simulink model "interpolation_cubique"  (R2017b)
settings: Solver=FixedStepDiscrete  StartTime=0.0  StopTime=1  RelTol=1e-3
model workspace (MAT data in the model file):
  bande_passante = 20000000
  binary_sample_time = 2.51968503937e-08
  display = [0+0i 0+0i 0+0i 0+0i 0+0i 0+0i 0+0i 0+0i 0+0i 0+0i 0+0i 0+0i ... (40000 elements, 200x200)]
  nbr_pilote = 3
  nbr_sous_porteuse = 508
  nbr_total_canaux = 512
  nbr_zero = 1
  size_prefixe_cyclique = 3
  symbol_sample_time = 2.56e-05
  v = [0+0i; 0+0i; 0+0i; 0+0i; 0+0i; 0+0i; 0+0i; 0+0i; 0+0i; 0+0i; 0+0i; 0+0i; 0+0i; 0+0i; 0+0i; 0+0i; 0+0i; 0+0i; 0+0i; 0+0i; 0+0i; 0+0i; 0+0i; 0+0i; 0+0i; 0+0i; 0+0i; 0+0i; 0+0i; 0+0i; 0+0i; 0+0i; 0+0i; 0+0i; 0+0i; 0+0i; 0+0i; 0+0i; 0+0i; 0+0i; 0+0i; 0+0i; 0+0i; 0+0i; 0+0i; 0+0i; 0+0i; 0+0i; 0+0i; 0+0i; 0+0i; 0+0i; 0+0i; 0+0i; 0+0i; 0+0i; 0+0i; 0+0i; 0+0i; 0+0i; 0+0i; 0+0i; 0+0i; 0+0i; 0+0i; 0+0i; 0+0i; 0+0i; 0+0i; 0+0i; 0+0i; 0+0i; 0+0i; 0+0i; 0+0i; 0+0i; 0+0i; 0+0i; 0+0i; 0+0i; 0+0i; 0+0i; 0+0i; 0+0i; 0+0i; 0+0i; 0+0i; 0+0i; 0+0i; 0+0i; 0+0i; 0+0i; 0+0i; 0+0i; 0+0i; 0+0i; 0+0i; 0+0i; 0+0i; 0+0i; 0+0i; 0+0i; 0+0i; 0+0i; 0+0i; 0+0i; 0+0i; 0+0i; 0+0i; 0+0i; 0+0i; 0+0i; 0+0i; 0+0i; 0+0i; 0+0i; 0+0i; 0+0i; 0+0i; 0+0i; 0+0i; 0+0i; 0+0i; 0+0i; 0+0i; 0+0i; 0+0i; 0+0i; 0+0i; 0+0i; 0+0i; 0+0i; 0+0i; 0+0i; 0+0i; 0+0i; 0+0i; 0+0i; 0+0i; 0+0i; 0+0i; 0+0i; 0+0i; 0+0i; 0+0i; 0+0i; 0+0i; 0+0i; 0+0i; 0+0i; 0+0i; 0+0i; 0+0i; 0+0i; 0+0i; 0+0i; 0+0i; 0+0i; 0+0i; 0+0i; 0+0i; 0+0i; 0+0i; 0+0i; 0+0i; 0+0i; 0+0i; 0+0i; 0+0i; 0+0i; 0+0i; 0+0i; 0+0i; 0+0i; 0+0i; 0+0i; 0+0i; 0+0i; 0+0i; 0+0i; 0+0i; 0+0i; 0+0i; 0+0i; 0+0i; 0+0i; 0+0i; 0+0i; 0+0i; 0+0i; 0+0i; 0+0i; 0+0i; 0+0i; 0+0i; 0+0i; 0+0i; 0+0i; 0+0i; 0+0i; 0+0i; 0+0i; 0+0i; 0+0i; 0+0i; 0+0i; 0+0i; 0+0i; 0+0i; 0+0i; 0+0i; 0+0i; 0+0i; 0+0i; 0+0i; 0+0i; 0+0i; 0+0i; 0+0i; 0+0i; 0+0i; 0+0i; 0+0i; 0+0i; 0+0i; 0+0i; 0+0i; 0+0i; 0+0i; 0+0i; 0+0i; 0+0i; 0+0i; 0+0i; 0+0i; 0+0i; 0+0i; 0+0i; 0+0i; 0+0i; 0+0i; 0+0i; 0+0i; 0+0i; 0+0i; 0+0i; 0+0i; 0+0i; 0+0i; 0+0i; 0+0i; 0+0i; 0+0i; 0+0i; 0+0i; 0+0i]
values from neighbouring files (symbols this model uses):
  interval_pilote = 150    [workspace.m]
undefined symbols (not defined in the file or in its folder): doppler
libraries: commchan3 x2, dspxfrm3 x2, dspindex x2, commdigbbndpm3 x2, commrandsrc3 x1, commsink2 x1
(part 1 of 2)
settings Model: SimulationMode=accelerator  Creator=jbblache  LastModifiedBy=hugy4
settings SolverCC: AutoInsertRateTranBlk=on
settings DataIOCC: LimitDataPoints=on  SaveOutput=off  SignalLogging=off  SaveTime=off
settings OptimizationCC: EfficientMapNaN2IntZero=off  LifeSpan=inf
settings DebuggingCC: AlgebraicLoopMsg=error  SingleTaskRateTransMsg=error  AllowSymbolicDim=off  SFUnexpectedBacktrackingDiag=warning  SFNoUnconditionalDefaultTransitionDiag=warning  SFExecutionAtInitializationDiag=none
settings HardwareCC: TargetBitPerPointer=64  TargetBitPerSizeT=64  TargetBitPerPtrDiffT=64  TargetLongLongMode=on  TargetIntDivRoundTo=Zero  TargetEndianess=LittleEndian  TargetWordSize=64  TargetHWDeviceType=MATLAB Host  ProdEqTarget=off
settings CodeAppCC: MaxIdLength=128
settings GRTTargetCC: TargetLangStandard=C89/C90 (ANSI)  CombineOutputUpdateFcns=off  GRTInterface=on

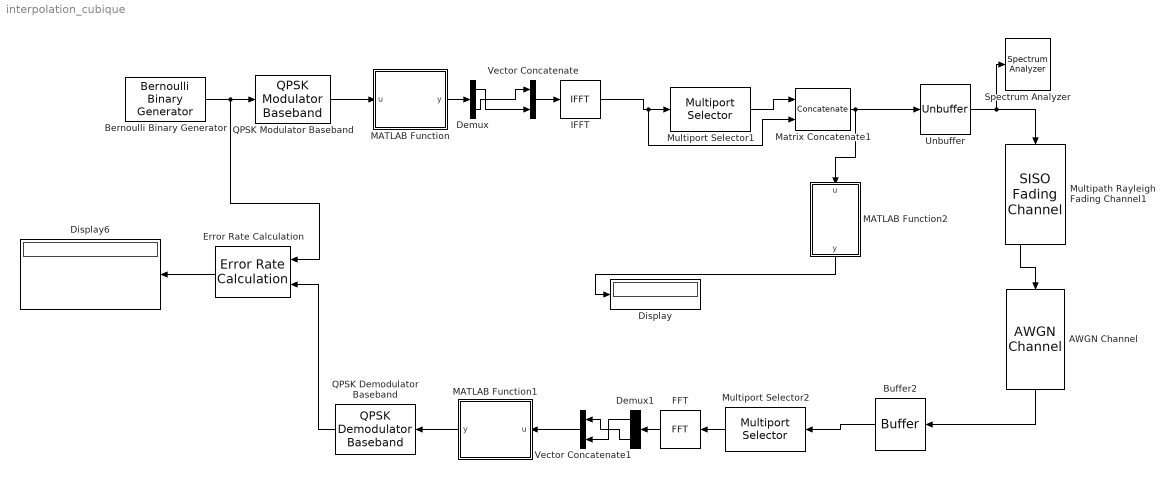
== system interpolation_cubique ==
  AWGN Channel : commchan3/AWGN Channel  InputProcessing=Columns as channels (frame based)  seed=67  noiseMode="Signal to noise ratio  (SNR)"  EbNodB=10  EsNodB=10  SNRdB=10  bitsPerSym=1  Ps=0.00195  Tsym=1  variance=1
  Bernoulli Binary Generator : commrandsrc3/Bernoulli Binary Generator  ProbabilityOfZero=0.5  SeedSource=Auto  Seed=0  SampleTime=binary_sample_time  SamplesPerFrame=nbr_sous_porteuse*2  OutputDataType=double  SimulateUsing=Interpreted execution
  Buffer2 : Buffer  N=nbr_total_canaux+size_prefixe_cyclique  OutputFrames=off
  Demux : Demux  Outputs=2
  Demux1 : Demux  Outputs=2
  Display : Display
  Display6 : Display
  Error Rate Calculation : commsink2/Error Rate Calculation  N=2 * nbr_sous_porteuse  st_delay=0  cp_mode=Entire frame  subframe=[]  PMode=Port  WsName=ErrorVec  RsMode2=off  stop=off  numErr=100  maxBits=1e6
  FFT : dspxfrm3/FFT  FFTImplementation=Auto  CompMethod=Table lookup  TableOpt=NEW  TableOptActive=Speed  BitRevOrder=off  Normalize=off  InheritFFTLength=on  FFTLength=64  WrapInput=off  roundingMode=Floor  overflowMode=off  firstCoeffDataTypeStr=Inherit: Same word length as input  firstCoeffLastDataTypeStr=Inherit: Same word length as input  outputMin=[]  outputMax=[]
  IFFT : dspxfrm3/IFFT  FFTImplementation=Auto  CompMethod=Table lookup  TableOpt=NEW  TableOptActive=Speed  BitRevOrder=off  cs_in=off  Normalize=on  InheritFFTLength=on  FFTLength=64  WrapInput=on  mode=Complex  outSamplingMode=Sample based  roundingMode=Floor  overflowMode=off  firstCoeffDataTypeStr=Inherit: Same word length as input  firstCoeffLastDataTypeStr=Inherit: Same word length as input  outputMin=[]  outputMax=[]
      settings: SourceProductName=DSP System Toolbox
  MATLAB Function : MATLAB Function  TreatAsAtomicUnit=on
  MATLAB Function1 : MATLAB Function  TreatAsAtomicUnit=on
  MATLAB Function2 : MATLAB Function  TreatAsAtomicUnit=on
  Matrix Concatenate1 : Concatenate  ConcatenateDimension=2
  Multipath Rayleigh Fading Channel1 : commchan3/SISO Fading Channel  PathDelays=[0 49.7087e-009 2*49.7087e-009]  AveragePathGains=[0 -3 -6]  NormalizePathGains=off  FadingDistribution=Rayleigh  KFactor=3  DirectPathDopplerShift=0  DirectPathInitialPhase=0  MaximumDopplerShift=0.001  DopplerSpectrum=doppler('Jakes')  RandomStream=mt19937ar with seed  RandomNumGenerator=shr3cong  Seed=73  PathGainsOutputPort=on  ChannelFilterDelayOutputPort=off  SimulateUsing=Interpreted execution  Visualization=Off  PathsForDopplerDisplay=1  SamplesToDisplay=25%
      settings: SourceProductName=Communications System Toolbox
  Multiport Selector1 : dspindex/Multiport Selector  rowsOrCols=Rows  idxCellArray={[nbr_total_canaux-(size_prefixe_cyclique-1):nbr_total_canaux] }  idxErrMode=Clip Index
  Multiport Selector2 : dspindex/Multiport Selector  rowsOrCols=Rows  idxCellArray={ [size_prefixe_cyclique+1:nbr_total_canaux+size_prefixe_cyclique] }  idxErrMode=Clip Index
  QPSK Demodulator Baseband : commdigbbndpm3/QPSK Demodulator Baseband  OutType=Bit  DecType=Hard decision  VarSource=Dialog  Variance=1  Dec=Gray  Ph=pi/4  outDtype1=Inherit via internal rule  outDtype2=Inherit via internal rule  derotateFactorWordLen=16  derotateFactorDataTypeStr=Inherit: Same word length as input  derotateFactorLastDataTypeStr=Inherit: Same word length as input
  QPSK Modulator Baseband : commdigbbndpm3/QPSK Modulator Baseband  InType=Bit  Enc=Gray  Ph=pi/4  outDtype=double  outWordLen=16  outUDDataType=sfix(16)  outFracLenMode=Best precision  outFracLen=15  outDataTypeStr=double  outLastDataTypeStr=double
  Spectrum Analyzer : SpectrumAnalyzer
  Unbuffer : Unbuffer
  Vector Concatenate : Concatenate
  Vector Concatenate1 : Concatenate
  wires:
  Bernoulli Binary Generator/1 -> Error Rate Calculation/1, QPSK Modulator Baseband/1
  QPSK Modulator Baseband/1 -> MATLAB Function/1(u)
  Multiport Selector1/1 -> Matrix Concatenate1/1
  MATLAB Function1/1(y) -> QPSK Demodulator Baseband/1
  QPSK Demodulator Baseband/1 -> Error Rate Calculation/2
  Buffer2/1 -> Multiport Selector2/1
  Unbuffer/1 -> Spectrum Analyzer/1, Multipath Rayleigh Fading Channel1/1
  AWGN Channel/1 -> Buffer2/1
  Multipath Rayleigh Fading Channel1/1 -> AWGN Channel/1
  Error Rate Calculation/1 -> Display6/1
  Matrix Concatenate1/1 -> MATLAB Function2/1(u), Unbuffer/1
  MATLAB Function2/1(y) -> Display/1
  IFFT/1 -> Matrix Concatenate1/2, Multiport Selector1/1
  MATLAB Function/1(y) -> Demux/1
  Demux/2 -> Vector Concatenate/1
  Demux/1 -> Vector Concatenate/2
  Vector Concatenate/1 -> IFFT/1
  Multiport Selector2/1 -> FFT/1
  Demux1/1 -> Vector Concatenate1/2
  Vector Concatenate1/1 -> MATLAB Function1/1(u)
  Demux1/2 -> Vector Concatenate1/1
  FFT/1 -> Demux1/1
